simulink library "AEMS_Standard_Library"  (R2016b)
settings: Solver=ode45  StartTime=0.0  StopTime=10.0  RelTol=1e-3
undefined symbols (not defined in the file or in its folder): BkPY, carto, Cbx_extegr, Cbx_lpegrsys, Cbx_portegr, Cnx_bnk_nr_conf, Cnx_cyl_nr_conf, ConfigManagement, configuration_management, Cxx_dcm_io_tmr_end_xxxx, Cxx_dcm_rt_tmr_end, Cxx_DID_xxxx_IO_max, Cxx_DID_xxxx_IO_min, Cxx_egrhsofs, Cxx_vmaniegi, DEM_DEBOUNCE_FREEZE, DEM_DTR_CTL_INVISIBLE, DEM_DTR_CTL_NORMAL, Dem_DtrId2_XXX, Dem_DtrId3_XXX, Dem_DtrId4_XXX, Dem_DtrId5_XXX, Dem_DtrId6_XXX, Dem_DtrId7_XXX, Dem_DtrId8_XXX, Dem_DtrId9_XXX, Dem_DtrId_XXX, Dem_EnableConditionId2_XXX, Dem_EnableConditionId3_XXX, Dem_EnableConditionId4_XXX, Dem_EnableConditionId5_XXX, Dem_EnableConditionId6_XXX, Dem_EnableConditionId7_XXX, Dem_EnableConditionId8_XXX, Dem_EnableConditionId_XXX, Dem_EventId, Dem_EventId2_XXX, Dem_EventId3_XXX, Dem_EventId4_XXX, Dem_EventId5_XXX, Dem_EventId6_XXX, Dem_EventId7_XXX, Dem_EventId8_XXX, Dem_EventId9_XXX, Dem_EventId_Device_Faulttype, Dem_EventId_XXX, DEM_IUMPR_GENERAL_DENOMINATOR, DEM_OPCYC_IGNITION, Dem_RatioId2_XXX, Dem_RatioId3_XXX, Dem_RatioId4_XXX, Dem_RatioId5_XXX, Dem_RatioId6_XXX, Dem_RatioId7_XXX, Dem_RatioId8_XXX, Dem_RatioId_XXX, Dem_StorageConditionId2_XXX, Dem_StorageConditionId3_XXX, Dem_StorageConditionId4_XXX, Dem_StorageConditionId5_XXX ... (+65)
libraries: AEMS_Standard_Library x477, simulink x2
(part 35 of 39)

== system AEMS_Standard_Library/SUB/AEMS_DEM_TIME_BASED_DEBOUNCE_8D/AEMS_DEM_TIME_BASED_DEBOUNCE_CALL8 ==
  conditionfulfilled : Inport
  prefailed : Inport  Port=2
  prepassed : Inport  Port=3
  reseteventdebounce : Inport  Port=4
  DemDebounceBehavior : Inport  Port=5
  DemCounterFailedThreshold : Inport  Port=6
  DemCounterPassedThreshold : Inport  Port=7
  Enable : EnablePort
  AEMS_DEM_TIMEBASEDDEBOUNCE : AEMS_Standard_Library/SUB/AEMS_DEM_TIMEBASEDDEBOUNCE  Tag=[LIB]  eventid=Dem_EventId_Device8_Faulttype  sampletime=0.01
      settings: AttributesFormatString=|
      | %<MaskType>
      | EventId: %<eventid>
      | Sample time: %<sampletime>
  debouncevalue_for_failed : Outport
  debouncevalue_for_passed : Outport  Port=2
  failed : Outport  Port=3
  passed : Outport  Port=4
  wires:
  DemCounterPassedThreshold/1 -> AEMS_DEM_TIMEBASEDDEBOUNCE/6
  DemDebounceBehavior/1 -> AEMS_DEM_TIMEBASEDDEBOUNCE/4
  conditionfulfilled/1 -> AEMS_DEM_TIMEBASEDDEBOUNCE/1
  prepassed/1 -> AEMS_DEM_TIMEBASEDDEBOUNCE/3
  reseteventdebounce/1 -> AEMS_DEM_TIMEBASEDDEBOUNCE/7
  prefailed/1 -> AEMS_DEM_TIMEBASEDDEBOUNCE/2
  DemCounterFailedThreshold/1 -> AEMS_DEM_TIMEBASEDDEBOUNCE/5
  AEMS_DEM_TIMEBASEDDEBOUNCE/1 -> debouncevalue_for_failed/1
  AEMS_DEM_TIMEBASEDDEBOUNCE/2 -> debouncevalue_for_passed/1
  AEMS_DEM_TIMEBASEDDEBOUNCE/3 -> failed/1
  AEMS_DEM_TIMEBASEDDEBOUNCE/4 -> passed/1

== system AEMS_Standard_Library/SUB/AEMS_DEM_TIME_BASED_DEBOUNCE_THRSHOLD_DYN_1D/AEMS_DEM_TIME_BASED_DEBOUNCE_THRSHOLD_DYN_CALL ==
  conditionfulfilled : Inport
  prefailed : Inport  Port=2
  prepassed : Inport  Port=3
  reseteventdebounce : Inport  Port=4
  DemDebounceBehavior : Inport  Port=5
  DemCounterFailedThreshold : Inport  Port=6
  DemCounterPassedThreshold : Inport  Port=7
  Enable : EnablePort
      settings: AttributesFormatString=StatesWhenEnabling = %<StatesWhenEnabling>
  AEMS_DEM_TIMEBASEDDEBOUNCE : AEMS_Standard_Library/SUB/AEMS_DEM_TIMEBASEDDEBOUNCE  Tag=[LIB]  eventid=Dem_EventId_Device_Faulttype  sampletime=0.01
      settings: AttributesFormatString=|
      | %<MaskType>
      | EventId: %<eventid>
      | Sample time: %<sampletime>
  debouncevalue_for_failed : Outport
      settings: AttributesFormatString=<initial=%<InitialOutput>>\n<whendisabled=%<OutputWhenDisabled>>
  debouncevalue_for_passed : Outport  Port=2
      settings: AttributesFormatString=<initial=%<InitialOutput>>\n<whendisabled=%<OutputWhenDisabled>>
  failed : Outport  Port=3
      settings: AttributesFormatString=<initial=%<InitialOutput>>\n<whendisabled=%<OutputWhenDisabled>>
  passed : Outport  Port=4
      settings: AttributesFormatString=<initial=%<InitialOutput>>\n<whendisabled=%<OutputWhenDisabled>>
  wires:
  AEMS_DEM_TIMEBASEDDEBOUNCE/4 -> passed/1
  AEMS_DEM_TIMEBASEDDEBOUNCE/3 -> failed/1
  AEMS_DEM_TIMEBASEDDEBOUNCE/2 -> debouncevalue_for_passed/1
  AEMS_DEM_TIMEBASEDDEBOUNCE/1 -> debouncevalue_for_failed/1
  DemCounterFailedThreshold/1 -> AEMS_DEM_TIMEBASEDDEBOUNCE/5
  prefailed/1 -> AEMS_DEM_TIMEBASEDDEBOUNCE/2
  reseteventdebounce/1 -> AEMS_DEM_TIMEBASEDDEBOUNCE/7
  prepassed/1 -> AEMS_DEM_TIMEBASEDDEBOUNCE/3
  conditionfulfilled/1 -> AEMS_DEM_TIMEBASEDDEBOUNCE/1
  DemDebounceBehavior/1 -> AEMS_DEM_TIMEBASEDDEBOUNCE/4
  DemCounterPassedThreshold/1 -> AEMS_DEM_TIMEBASEDDEBOUNCE/6

== system AEMS_Standard_Library/SUB/AEMS_DEM_TIME_BASED_DEBOUNCE_THRSHOLD_DYN_2D/AEMS_DEM_TIME_BASED_DEBOUNCE_THRSHOLD_DYN_CALL1 ==
  conditionfulfilled : Inport
  prefailed : Inport  Port=2
  prepassed : Inport  Port=3
  reseteventdebounce : Inport  Port=4
  DemDebounceBehavior : Inport  Port=5
  DemCounterFailedThreshold : Inport  Port=6
  DemCounterPassedThreshold : Inport  Port=7
  Enable : EnablePort
      settings: AttributesFormatString=StatesWhenEnabling = %<StatesWhenEnabling>
  AEMS_DEM_TIMEBASEDDEBOUNCE : AEMS_Standard_Library/SUB/AEMS_DEM_TIMEBASEDDEBOUNCE  Tag=[LIB]  eventid=Dem_EventId_Device_Faulttype  sampletime=0.01
      settings: AttributesFormatString=|
      | %<MaskType>
      | EventId: %<eventid>
      | Sample time: %<sampletime>
  debouncevalue_for_failed : Outport
      settings: AttributesFormatString=<initial=%<InitialOutput>>\n<whendisabled=%<OutputWhenDisabled>>
  debouncevalue_for_passed : Outport  Port=2
      settings: AttributesFormatString=<initial=%<InitialOutput>>\n<whendisabled=%<OutputWhenDisabled>>
  failed : Outport  Port=3
      settings: AttributesFormatString=<initial=%<InitialOutput>>\n<whendisabled=%<OutputWhenDisabled>>
  passed : Outport  Port=4
      settings: AttributesFormatString=<initial=%<InitialOutput>>\n<whendisabled=%<OutputWhenDisabled>>
  wires:
  AEMS_DEM_TIMEBASEDDEBOUNCE/4 -> passed/1
  AEMS_DEM_TIMEBASEDDEBOUNCE/3 -> failed/1
  AEMS_DEM_TIMEBASEDDEBOUNCE/2 -> debouncevalue_for_passed/1
  AEMS_DEM_TIMEBASEDDEBOUNCE/1 -> debouncevalue_for_failed/1
  DemCounterFailedThreshold/1 -> AEMS_DEM_TIMEBASEDDEBOUNCE/5
  prefailed/1 -> AEMS_DEM_TIMEBASEDDEBOUNCE/2
  reseteventdebounce/1 -> AEMS_DEM_TIMEBASEDDEBOUNCE/7
  prepassed/1 -> AEMS_DEM_TIMEBASEDDEBOUNCE/3
  conditionfulfilled/1 -> AEMS_DEM_TIMEBASEDDEBOUNCE/1
  DemDebounceBehavior/1 -> AEMS_DEM_TIMEBASEDDEBOUNCE/4
  DemCounterPassedThreshold/1 -> AEMS_DEM_TIMEBASEDDEBOUNCE/6

== system AEMS_Standard_Library/SUB/AEMS_DEM_TIME_BASED_DEBOUNCE_THRSHOLD_DYN_2D/AEMS_DEM_TIME_BASED_DEBOUNCE_THRSHOLD_DYN_CALL2 ==
  conditionfulfilled : Inport
  prefailed : Inport  Port=2
  prepassed : Inport  Port=3
  reseteventdebounce : Inport  Port=4
  DemDebounceBehavior : Inport  Port=5
  DemCounterFailedThreshold : Inport  Port=6
  DemCounterPassedThreshold : Inport  Port=7
  Enable : EnablePort
      settings: AttributesFormatString=StatesWhenEnabling = %<StatesWhenEnabling>
  AEMS_DEM_TIMEBASEDDEBOUNCE : AEMS_Standard_Library/SUB/AEMS_DEM_TIMEBASEDDEBOUNCE  Tag=[LIB]  eventid=Dem_EventId_Device2_Faulttype  sampletime=0.01
      settings: AttributesFormatString=|
      | %<MaskType>
      | EventId: %<eventid>
      | Sample time: %<sampletime>
  debouncevalue_for_failed : Outport
      settings: AttributesFormatString=<initial=%<InitialOutput>>\n<whendisabled=%<OutputWhenDisabled>>
  debouncevalue_for_passed : Outport  Port=2
      settings: AttributesFormatString=<initial=%<InitialOutput>>\n<whendisabled=%<OutputWhenDisabled>>
  failed : Outport  Port=3
      settings: AttributesFormatString=<initial=%<InitialOutput>>\n<whendisabled=%<OutputWhenDisabled>>
  passed : Outport  Port=4
      settings: AttributesFormatString=<initial=%<InitialOutput>>\n<whendisabled=%<OutputWhenDisabled>>
  wires:
  DemCounterPassedThreshold/1 -> AEMS_DEM_TIMEBASEDDEBOUNCE/6
  DemDebounceBehavior/1 -> AEMS_DEM_TIMEBASEDDEBOUNCE/4
  conditionfulfilled/1 -> AEMS_DEM_TIMEBASEDDEBOUNCE/1
  prepassed/1 -> AEMS_DEM_TIMEBASEDDEBOUNCE/3
  reseteventdebounce/1 -> AEMS_DEM_TIMEBASEDDEBOUNCE/7
  prefailed/1 -> AEMS_DEM_TIMEBASEDDEBOUNCE/2
  DemCounterFailedThreshold/1 -> AEMS_DEM_TIMEBASEDDEBOUNCE/5
  AEMS_DEM_TIMEBASEDDEBOUNCE/1 -> debouncevalue_for_failed/1
  AEMS_DEM_TIMEBASEDDEBOUNCE/2 -> debouncevalue_for_passed/1
  AEMS_DEM_TIMEBASEDDEBOUNCE/3 -> failed/1
  AEMS_DEM_TIMEBASEDDEBOUNCE/4 -> passed/1

== system AEMS_Standard_Library/SUB/AEMS_DEM_TIME_BASED_DEBOUNCE_THRSHOLD_DYN_3D/AEMS_DEM_TIME_BASED_DEBOUNCE_THRSHOLD_DYN_CALL1 ==
  conditionfulfilled : Inport
  prefailed : Inport  Port=2
  prepassed : Inport  Port=3
  reseteventdebounce : Inport  Port=4
  DemDebounceBehavior : Inport  Port=5
  DemCounterFailedThreshold : Inport  Port=6
  DemCounterPassedThreshold : Inport  Port=7
  Enable : EnablePort
      settings: AttributesFormatString=StatesWhenEnabling = %<StatesWhenEnabling>
  AEMS_DEM_TIMEBASEDDEBOUNCE : AEMS_Standard_Library/SUB/AEMS_DEM_TIMEBASEDDEBOUNCE  Tag=[LIB]  eventid=Dem_EventId_Device_Faulttype  sampletime=0.01
      settings: AttributesFormatString=|
      | %<MaskType>
      | EventId: %<eventid>
      | Sample time: %<sampletime>
  debouncevalue_for_failed : Outport
      settings: AttributesFormatString=<initial=%<InitialOutput>>\n<whendisabled=%<OutputWhenDisabled>>
  debouncevalue_for_passed : Outport  Port=2
      settings: AttributesFormatString=<initial=%<InitialOutput>>\n<whendisabled=%<OutputWhenDisabled>>
  failed : Outport  Port=3
      settings: AttributesFormatString=<initial=%<InitialOutput>>\n<whendisabled=%<OutputWhenDisabled>>
  passed : Outport  Port=4
      settings: AttributesFormatString=<initial=%<InitialOutput>>\n<whendisabled=%<OutputWhenDisabled>>
  wires:
  AEMS_DEM_TIMEBASEDDEBOUNCE/4 -> passed/1
  AEMS_DEM_TIMEBASEDDEBOUNCE/3 -> failed/1
  AEMS_DEM_TIMEBASEDDEBOUNCE/2 -> debouncevalue_for_passed/1
  AEMS_DEM_TIMEBASEDDEBOUNCE/1 -> debouncevalue_for_failed/1
  DemCounterFailedThreshold/1 -> AEMS_DEM_TIMEBASEDDEBOUNCE/5
  prefailed/1 -> AEMS_DEM_TIMEBASEDDEBOUNCE/2
  reseteventdebounce/1 -> AEMS_DEM_TIMEBASEDDEBOUNCE/7
  prepassed/1 -> AEMS_DEM_TIMEBASEDDEBOUNCE/3
  conditionfulfilled/1 -> AEMS_DEM_TIMEBASEDDEBOUNCE/1
  DemDebounceBehavior/1 -> AEMS_DEM_TIMEBASEDDEBOUNCE/4
  DemCounterPassedThreshold/1 -> AEMS_DEM_TIMEBASEDDEBOUNCE/6

== system AEMS_Standard_Library/SUB/AEMS_DEM_TIME_BASED_DEBOUNCE_THRSHOLD_DYN_3D/AEMS_DEM_TIME_BASED_DEBOUNCE_THRSHOLD_DYN_CALL2 ==
  conditionfulfilled : Inport
  prefailed : Inport  Port=2
  prepassed : Inport  Port=3
  reseteventdebounce : Inport  Port=4
  DemDebounceBehavior : Inport  Port=5
  DemCounterFailedThreshold : Inport  Port=6
  DemCounterPassedThreshold : Inport  Port=7
  Enable : EnablePort
      settings: AttributesFormatString=StatesWhenEnabling = %<StatesWhenEnabling>
  AEMS_DEM_TIMEBASEDDEBOUNCE : AEMS_Standard_Library/SUB/AEMS_DEM_TIMEBASEDDEBOUNCE  Tag=[LIB]  eventid=Dem_EventId_Device2_Faulttype  sampletime=0.01
      settings: AttributesFormatString=|
      | %<MaskType>
      | EventId: %<eventid>
      | Sample time: %<sampletime>
  debouncevalue_for_failed : Outport
      settings: AttributesFormatString=<initial=%<InitialOutput>>\n<whendisabled=%<OutputWhenDisabled>>
  debouncevalue_for_passed : Outport  Port=2
      settings: AttributesFormatString=<initial=%<InitialOutput>>\n<whendisabled=%<OutputWhenDisabled>>
  failed : Outport  Port=3
      settings: AttributesFormatString=<initial=%<InitialOutput>>\n<whendisabled=%<OutputWhenDisabled>>
  passed : Outport  Port=4
      settings: AttributesFormatString=<initial=%<InitialOutput>>\n<whendisabled=%<OutputWhenDisabled>>
  wires:
  DemCounterPassedThreshold/1 -> AEMS_DEM_TIMEBASEDDEBOUNCE/6
  DemDebounceBehavior/1 -> AEMS_DEM_TIMEBASEDDEBOUNCE/4
  conditionfulfilled/1 -> AEMS_DEM_TIMEBASEDDEBOUNCE/1
  prepassed/1 -> AEMS_DEM_TIMEBASEDDEBOUNCE/3
  reseteventdebounce/1 -> AEMS_DEM_TIMEBASEDDEBOUNCE/7
  prefailed/1 -> AEMS_DEM_TIMEBASEDDEBOUNCE/2
  DemCounterFailedThreshold/1 -> AEMS_DEM_TIMEBASEDDEBOUNCE/5
  AEMS_DEM_TIMEBASEDDEBOUNCE/1 -> debouncevalue_for_failed/1
  AEMS_DEM_TIMEBASEDDEBOUNCE/2 -> debouncevalue_for_passed/1
  AEMS_DEM_TIMEBASEDDEBOUNCE/3 -> failed/1
  AEMS_DEM_TIMEBASEDDEBOUNCE/4 -> passed/1

== system AEMS_Standard_Library/SUB/AEMS_DEM_TIME_BASED_DEBOUNCE_THRSHOLD_DYN_3D/AEMS_DEM_TIME_BASED_DEBOUNCE_THRSHOLD_DYN_CALL3 ==
  conditionfulfilled : Inport
  prefailed : Inport  Port=2
  prepassed : Inport  Port=3
  reseteventdebounce : Inport  Port=4
  DemDebounceBehavior : Inport  Port=5
  DemCounterFailedThreshold : Inport  Port=6
  DemCounterPassedThreshold : Inport  Port=7
  Enable : EnablePort
      settings: AttributesFormatString=StatesWhenEnabling = %<StatesWhenEnabling>
  AEMS_DEM_TIMEBASEDDEBOUNCE : AEMS_Standard_Library/SUB/AEMS_DEM_TIMEBASEDDEBOUNCE  Tag=[LIB]  eventid=Dem_EventId_Device3_Faulttype  sampletime=0.01
      settings: AttributesFormatString=|
      | %<MaskType>
      | EventId: %<eventid>
      | Sample time: %<sampletime>
  debouncevalue_for_failed : Outport
      settings: AttributesFormatString=<initial=%<InitialOutput>>\n<whendisabled=%<OutputWhenDisabled>>
  debouncevalue_for_passed : Outport  Port=2
      settings: AttributesFormatString=<initial=%<InitialOutput>>\n<whendisabled=%<OutputWhenDisabled>>
  failed : Outport  Port=3
      settings: AttributesFormatString=<initial=%<InitialOutput>>\n<whendisabled=%<OutputWhenDisabled>>
  passed : Outport  Port=4
      settings: AttributesFormatString=<initial=%<InitialOutput>>\n<whendisabled=%<OutputWhenDisabled>>
  wires:
  DemCounterPassedThreshold/1 -> AEMS_DEM_TIMEBASEDDEBOUNCE/6
  DemDebounceBehavior/1 -> AEMS_DEM_TIMEBASEDDEBOUNCE/4
  conditionfulfilled/1 -> AEMS_DEM_TIMEBASEDDEBOUNCE/1
  prepassed/1 -> AEMS_DEM_TIMEBASEDDEBOUNCE/3
  reseteventdebounce/1 -> AEMS_DEM_TIMEBASEDDEBOUNCE/7
  prefailed/1 -> AEMS_DEM_TIMEBASEDDEBOUNCE/2
  DemCounterFailedThreshold/1 -> AEMS_DEM_TIMEBASEDDEBOUNCE/5
  AEMS_DEM_TIMEBASEDDEBOUNCE/1 -> debouncevalue_for_failed/1
  AEMS_DEM_TIMEBASEDDEBOUNCE/2 -> debouncevalue_for_passed/1
  AEMS_DEM_TIMEBASEDDEBOUNCE/3 -> failed/1
  AEMS_DEM_TIMEBASEDDEBOUNCE/4 -> passed/1

== system AEMS_Standard_Library/SUB/AEMS_DEM_TIME_BASED_DEBOUNCE_THRSHOLD_DYN_4D/AEMS_DEM_TIME_BASED_DEBOUNCE_THRSHOLD_DYN_CALL1 ==
  conditionfulfilled : Inport
  prefailed : Inport  Port=2
  prepassed : Inport  Port=3
  reseteventdebounce : Inport  Port=4
  DemDebounceBehavior : Inport  Port=5
  DemCounterFailedThreshold : Inport  Port=6
  DemCounterPassedThreshold : Inport  Port=7
  Enable : EnablePort
      settings: AttributesFormatString=StatesWhenEnabling = %<StatesWhenEnabling>
  AEMS_DEM_TIMEBASEDDEBOUNCE : AEMS_Standard_Library/SUB/AEMS_DEM_TIMEBASEDDEBOUNCE  Tag=[LIB]  eventid=Dem_EventId_Device_Faulttype  sampletime=0.01
      settings: AttributesFormatString=|
      | %<MaskType>
      | EventId: %<eventid>
      | Sample time: %<sampletime>
  debouncevalue_for_failed : Outport
      settings: AttributesFormatString=<initial=%<InitialOutput>>\n<whendisabled=%<OutputWhenDisabled>>
  debouncevalue_for_passed : Outport  Port=2
      settings: AttributesFormatString=<initial=%<InitialOutput>>\n<whendisabled=%<OutputWhenDisabled>>
  failed : Outport  Port=3
      settings: AttributesFormatString=<initial=%<InitialOutput>>\n<whendisabled=%<OutputWhenDisabled>>
  passed : Outport  Port=4
      settings: AttributesFormatString=<initial=%<InitialOutput>>\n<whendisabled=%<OutputWhenDisabled>>
  wires:
  AEMS_DEM_TIMEBASEDDEBOUNCE/4 -> passed/1
  AEMS_DEM_TIMEBASEDDEBOUNCE/3 -> failed/1
  AEMS_DEM_TIMEBASEDDEBOUNCE/2 -> debouncevalue_for_passed/1
  AEMS_DEM_TIMEBASEDDEBOUNCE/1 -> debouncevalue_for_failed/1
  DemCounterFailedThreshold/1 -> AEMS_DEM_TIMEBASEDDEBOUNCE/5
  prefailed/1 -> AEMS_DEM_TIMEBASEDDEBOUNCE/2
  reseteventdebounce/1 -> AEMS_DEM_TIMEBASEDDEBOUNCE/7
  prepassed/1 -> AEMS_DEM_TIMEBASEDDEBOUNCE/3
  conditionfulfilled/1 -> AEMS_DEM_TIMEBASEDDEBOUNCE/1
  DemDebounceBehavior/1 -> AEMS_DEM_TIMEBASEDDEBOUNCE/4
  DemCounterPassedThreshold/1 -> AEMS_DEM_TIMEBASEDDEBOUNCE/6

== system AEMS_Standard_Library/SUB/AEMS_DEM_TIME_BASED_DEBOUNCE_THRSHOLD_DYN_4D/AEMS_DEM_TIME_BASED_DEBOUNCE_THRSHOLD_DYN_CALL2 ==
  conditionfulfilled : Inport
  prefailed : Inport  Port=2
  prepassed : Inport  Port=3
  reseteventdebounce : Inport  Port=4
  DemDebounceBehavior : Inport  Port=5
  DemCounterFailedThreshold : Inport  Port=6
  DemCounterPassedThreshold : Inport  Port=7
  Enable : EnablePort
      settings: AttributesFormatString=StatesWhenEnabling = %<StatesWhenEnabling>
  AEMS_DEM_TIMEBASEDDEBOUNCE : AEMS_Standard_Library/SUB/AEMS_DEM_TIMEBASEDDEBOUNCE  Tag=[LIB]  eventid=Dem_EventId_Device2_Faulttype  sampletime=0.01
      settings: AttributesFormatString=|
      | %<MaskType>
      | EventId: %<eventid>
      | Sample time: %<sampletime>
  debouncevalue_for_failed : Outport
      settings: AttributesFormatString=<initial=%<InitialOutput>>\n<whendisabled=%<OutputWhenDisabled>>
  debouncevalue_for_passed : Outport  Port=2
      settings: AttributesFormatString=<initial=%<InitialOutput>>\n<whendisabled=%<OutputWhenDisabled>>
  failed : Outport  Port=3
      settings: AttributesFormatString=<initial=%<InitialOutput>>\n<whendisabled=%<OutputWhenDisabled>>
  passed : Outport  Port=4
      settings: AttributesFormatString=<initial=%<InitialOutput>>\n<whendisabled=%<OutputWhenDisabled>>
  wires:
  DemCounterPassedThreshold/1 -> AEMS_DEM_TIMEBASEDDEBOUNCE/6
  DemDebounceBehavior/1 -> AEMS_DEM_TIMEBASEDDEBOUNCE/4
  conditionfulfilled/1 -> AEMS_DEM_TIMEBASEDDEBOUNCE/1
  prepassed/1 -> AEMS_DEM_TIMEBASEDDEBOUNCE/3
  reseteventdebounce/1 -> AEMS_DEM_TIMEBASEDDEBOUNCE/7
  prefailed/1 -> AEMS_DEM_TIMEBASEDDEBOUNCE/2
  DemCounterFailedThreshold/1 -> AEMS_DEM_TIMEBASEDDEBOUNCE/5
  AEMS_DEM_TIMEBASEDDEBOUNCE/1 -> debouncevalue_for_failed/1
  AEMS_DEM_TIMEBASEDDEBOUNCE/2 -> debouncevalue_for_passed/1
  AEMS_DEM_TIMEBASEDDEBOUNCE/3 -> failed/1
  AEMS_DEM_TIMEBASEDDEBOUNCE/4 -> passed/1

== system AEMS_Standard_Library/SUB/AEMS_DEM_TIME_BASED_DEBOUNCE_THRSHOLD_DYN_4D/AEMS_DEM_TIME_BASED_DEBOUNCE_THRSHOLD_DYN_CALL3 ==
  conditionfulfilled : Inport
  prefailed : Inport  Port=2
  prepassed : Inport  Port=3
  reseteventdebounce : Inport  Port=4
  DemDebounceBehavior : Inport  Port=5
  DemCounterFailedThreshold : Inport  Port=6
  DemCounterPassedThreshold : Inport  Port=7
  Enable : EnablePort
      settings: AttributesFormatString=StatesWhenEnabling = %<StatesWhenEnabling>
  AEMS_DEM_TIMEBASEDDEBOUNCE : AEMS_Standard_Library/SUB/AEMS_DEM_TIMEBASEDDEBOUNCE  Tag=[LIB]  eventid=Dem_EventId_Device3_Faulttype  sampletime=0.01
      settings: AttributesFormatString=|
      | %<MaskType>
      | EventId: %<eventid>
      | Sample time: %<sampletime>
  debouncevalue_for_failed : Outport
      settings: AttributesFormatString=<initial=%<InitialOutput>>\n<whendisabled=%<OutputWhenDisabled>>
  debouncevalue_for_passed : Outport  Port=2
      settings: AttributesFormatString=<initial=%<InitialOutput>>\n<whendisabled=%<OutputWhenDisabled>>
  failed : Outport  Port=3
      settings: AttributesFormatString=<initial=%<InitialOutput>>\n<whendisabled=%<OutputWhenDisabled>>
  passed : Outport  Port=4
      settings: AttributesFormatString=<initial=%<InitialOutput>>\n<whendisabled=%<OutputWhenDisabled>>
  wires:
  DemCounterPassedThreshold/1 -> AEMS_DEM_TIMEBASEDDEBOUNCE/6
  DemDebounceBehavior/1 -> AEMS_DEM_TIMEBASEDDEBOUNCE/4
  conditionfulfilled/1 -> AEMS_DEM_TIMEBASEDDEBOUNCE/1
  prepassed/1 -> AEMS_DEM_TIMEBASEDDEBOUNCE/3
  reseteventdebounce/1 -> AEMS_DEM_TIMEBASEDDEBOUNCE/7
  prefailed/1 -> AEMS_DEM_TIMEBASEDDEBOUNCE/2
  DemCounterFailedThreshold/1 -> AEMS_DEM_TIMEBASEDDEBOUNCE/5
  AEMS_DEM_TIMEBASEDDEBOUNCE/1 -> debouncevalue_for_failed/1
  AEMS_DEM_TIMEBASEDDEBOUNCE/2 -> debouncevalue_for_passed/1
  AEMS_DEM_TIMEBASEDDEBOUNCE/3 -> failed/1
  AEMS_DEM_TIMEBASEDDEBOUNCE/4 -> passed/1

== system AEMS_Standard_Library/SUB/AEMS_DEM_TIME_BASED_DEBOUNCE_THRSHOLD_DYN_4D/AEMS_DEM_TIME_BASED_DEBOUNCE_THRSHOLD_DYN_CALL4 ==
  conditionfulfilled : Inport
  prefailed : Inport  Port=2
  prepassed : Inport  Port=3
  reseteventdebounce : Inport  Port=4
  DemDebounceBehavior : Inport  Port=5
  DemCounterFailedThreshold : Inport  Port=6
  DemCounterPassedThreshold : Inport  Port=7
  Enable : EnablePort
      settings: AttributesFormatString=StatesWhenEnabling = %<StatesWhenEnabling>
  AEMS_DEM_TIMEBASEDDEBOUNCE : AEMS_Standard_Library/SUB/AEMS_DEM_TIMEBASEDDEBOUNCE  Tag=[LIB]  eventid=Dem_EventId_Device4_Faulttype  sampletime=0.01
      settings: AttributesFormatString=|
      | %<MaskType>
      | EventId: %<eventid>
      | Sample time: %<sampletime>
  debouncevalue_for_failed : Outport
      settings: AttributesFormatString=<initial=%<InitialOutput>>\n<whendisabled=%<OutputWhenDisabled>>
  debouncevalue_for_passed : Outport  Port=2
      settings: AttributesFormatString=<initial=%<InitialOutput>>\n<whendisabled=%<OutputWhenDisabled>>
  failed : Outport  Port=3
      settings: AttributesFormatString=<initial=%<InitialOutput>>\n<whendisabled=%<OutputWhenDisabled>>
  passed : Outport  Port=4
      settings: AttributesFormatString=<initial=%<InitialOutput>>\n<whendisabled=%<OutputWhenDisabled>>
  wires:
  DemCounterPassedThreshold/1 -> AEMS_DEM_TIMEBASEDDEBOUNCE/6
  DemDebounceBehavior/1 -> AEMS_DEM_TIMEBASEDDEBOUNCE/4
  conditionfulfilled/1 -> AEMS_DEM_TIMEBASEDDEBOUNCE/1
  prepassed/1 -> AEMS_DEM_TIMEBASEDDEBOUNCE/3
  reseteventdebounce/1 -> AEMS_DEM_TIMEBASEDDEBOUNCE/7
  prefailed/1 -> AEMS_DEM_TIMEBASEDDEBOUNCE/2
  DemCounterFailedThreshold/1 -> AEMS_DEM_TIMEBASEDDEBOUNCE/5
  AEMS_DEM_TIMEBASEDDEBOUNCE/1 -> debouncevalue_for_failed/1
  AEMS_DEM_TIMEBASEDDEBOUNCE/2 -> debouncevalue_for_passed/1
  AEMS_DEM_TIMEBASEDDEBOUNCE/3 -> failed/1
  AEMS_DEM_TIMEBASEDDEBOUNCE/4 -> passed/1

== system AEMS_Standard_Library/SUB/AEMS_DEM_TIME_BASED_DEBOUNCE_THRSHOLD_DYN_6D/AEMS_DEM_TIME_BASED_DEBOUNCE_THRSHOLD_DYN_CALL1 ==
  conditionfulfilled : Inport
  prefailed : Inport  Port=2
  prepassed : Inport  Port=3
  reseteventdebounce : Inport  Port=4
  DemDebounceBehavior : Inport  Port=5
  DemCounterFailedThreshold : Inport  Port=6
  DemCounterPassedThreshold : Inport  Port=7
  Enable : EnablePort
      settings: AttributesFormatString=StatesWhenEnabling = %<StatesWhenEnabling>
  AEMS_DEM_TIMEBASEDDEBOUNCE : AEMS_Standard_Library/SUB/AEMS_DEM_TIMEBASEDDEBOUNCE  Tag=[LIB]  eventid=Dem_EventId_Device_Faulttype  sampletime=0.01
      settings: AttributesFormatString=|
      | %<MaskType>
      | EventId: %<eventid>
      | Sample time: %<sampletime>
  debouncevalue_for_failed : Outport
      settings: AttributesFormatString=<initial=%<InitialOutput>>\n<whendisabled=%<OutputWhenDisabled>>
  debouncevalue_for_passed : Outport  Port=2
      settings: AttributesFormatString=<initial=%<InitialOutput>>\n<whendisabled=%<OutputWhenDisabled>>
  failed : Outport  Port=3
      settings: AttributesFormatString=<initial=%<InitialOutput>>\n<whendisabled=%<OutputWhenDisabled>>
  passed : Outport  Port=4
      settings: AttributesFormatString=<initial=%<InitialOutput>>\n<whendisabled=%<OutputWhenDisabled>>
  wires:
  DemCounterPassedThreshold/1 -> AEMS_DEM_TIMEBASEDDEBOUNCE/6
  DemDebounceBehavior/1 -> AEMS_DEM_TIMEBASEDDEBOUNCE/4
  conditionfulfilled/1 -> AEMS_DEM_TIMEBASEDDEBOUNCE/1
  prepassed/1 -> AEMS_DEM_TIMEBASEDDEBOUNCE/3
  reseteventdebounce/1 -> AEMS_DEM_TIMEBASEDDEBOUNCE/7
  prefailed/1 -> AEMS_DEM_TIMEBASEDDEBOUNCE/2
  DemCounterFailedThreshold/1 -> AEMS_DEM_TIMEBASEDDEBOUNCE/5
  AEMS_DEM_TIMEBASEDDEBOUNCE/1 -> debouncevalue_for_failed/1
  AEMS_DEM_TIMEBASEDDEBOUNCE/2 -> debouncevalue_for_passed/1
  AEMS_DEM_TIMEBASEDDEBOUNCE/3 -> failed/1
  AEMS_DEM_TIMEBASEDDEBOUNCE/4 -> passed/1

== system AEMS_Standard_Library/SUB/AEMS_DEM_TIME_BASED_DEBOUNCE_THRSHOLD_DYN_6D/AEMS_DEM_TIME_BASED_DEBOUNCE_THRSHOLD_DYN_CALL2 ==
  conditionfulfilled : Inport
  prefailed : Inport  Port=2
  prepassed : Inport  Port=3
  reseteventdebounce : Inport  Port=4
  DemDebounceBehavior : Inport  Port=5
  DemCounterFailedThreshold : Inport  Port=6
  DemCounterPassedThreshold : Inport  Port=7
  Enable : EnablePort
      settings: AttributesFormatString=StatesWhenEnabling = %<StatesWhenEnabling>
  AEMS_DEM_TIMEBASEDDEBOUNCE : AEMS_Standard_Library/SUB/AEMS_DEM_TIMEBASEDDEBOUNCE  Tag=[LIB]  eventid=Dem_EventId_Device2_Faulttype  sampletime=0.01
      settings: AttributesFormatString=|
      | %<MaskType>
      | EventId: %<eventid>
      | Sample time: %<sampletime>
  debouncevalue_for_failed : Outport
      settings: AttributesFormatString=<initial=%<InitialOutput>>\n<whendisabled=%<OutputWhenDisabled>>
  debouncevalue_for_passed : Outport  Port=2
      settings: AttributesFormatString=<initial=%<InitialOutput>>\n<whendisabled=%<OutputWhenDisabled>>
  failed : Outport  Port=3
      settings: AttributesFormatString=<initial=%<InitialOutput>>\n<whendisabled=%<OutputWhenDisabled>>
  passed : Outport  Port=4
      settings: AttributesFormatString=<initial=%<InitialOutput>>\n<whendisabled=%<OutputWhenDisabled>>
  wires:
  AEMS_DEM_TIMEBASEDDEBOUNCE/4 -> passed/1
  AEMS_DEM_TIMEBASEDDEBOUNCE/3 -> failed/1
  AEMS_DEM_TIMEBASEDDEBOUNCE/2 -> debouncevalue_for_passed/1
  AEMS_DEM_TIMEBASEDDEBOUNCE/1 -> debouncevalue_for_failed/1
  DemCounterFailedThreshold/1 -> AEMS_DEM_TIMEBASEDDEBOUNCE/5
  prefailed/1 -> AEMS_DEM_TIMEBASEDDEBOUNCE/2
  reseteventdebounce/1 -> AEMS_DEM_TIMEBASEDDEBOUNCE/7
  prepassed/1 -> AEMS_DEM_TIMEBASEDDEBOUNCE/3
  conditionfulfilled/1 -> AEMS_DEM_TIMEBASEDDEBOUNCE/1
  DemDebounceBehavior/1 -> AEMS_DEM_TIMEBASEDDEBOUNCE/4
  DemCounterPassedThreshold/1 -> AEMS_DEM_TIMEBASEDDEBOUNCE/6

== system AEMS_Standard_Library/SUB/AEMS_DEM_TIME_BASED_DEBOUNCE_THRSHOLD_DYN_6D/AEMS_DEM_TIME_BASED_DEBOUNCE_THRSHOLD_DYN_CALL3 ==
  conditionfulfilled : Inport
  prefailed : Inport  Port=2
  prepassed : Inport  Port=3
  reseteventdebounce : Inport  Port=4
  DemDebounceBehavior : Inport  Port=5
  DemCounterFailedThreshold : Inport  Port=6
  DemCounterPassedThreshold : Inport  Port=7
  Enable : EnablePort
      settings: AttributesFormatString=StatesWhenEnabling = %<StatesWhenEnabling>
  AEMS_DEM_TIMEBASEDDEBOUNCE : AEMS_Standard_Library/SUB/AEMS_DEM_TIMEBASEDDEBOUNCE  Tag=[LIB]  eventid=Dem_EventId_Device3_Faulttype  sampletime=0.01
      settings: AttributesFormatString=|
      | %<MaskType>
      | EventId: %<eventid>
      | Sample time: %<sampletime>
  debouncevalue_for_failed : Outport
      settings: AttributesFormatString=<initial=%<InitialOutput>>\n<whendisabled=%<OutputWhenDisabled>>
  debouncevalue_for_passed : Outport  Port=2
      settings: AttributesFormatString=<initial=%<InitialOutput>>\n<whendisabled=%<OutputWhenDisabled>>
  failed : Outport  Port=3
      settings: AttributesFormatString=<initial=%<InitialOutput>>\n<whendisabled=%<OutputWhenDisabled>>
  passed : Outport  Port=4
      settings: AttributesFormatString=<initial=%<InitialOutput>>\n<whendisabled=%<OutputWhenDisabled>>
  wires:
  AEMS_DEM_TIMEBASEDDEBOUNCE/4 -> passed/1
  AEMS_DEM_TIMEBASEDDEBOUNCE/3 -> failed/1
  AEMS_DEM_TIMEBASEDDEBOUNCE/2 -> debouncevalue_for_passed/1
  AEMS_DEM_TIMEBASEDDEBOUNCE/1 -> debouncevalue_for_failed/1
  DemCounterFailedThreshold/1 -> AEMS_DEM_TIMEBASEDDEBOUNCE/5
  prefailed/1 -> AEMS_DEM_TIMEBASEDDEBOUNCE/2
  reseteventdebounce/1 -> AEMS_DEM_TIMEBASEDDEBOUNCE/7
  prepassed/1 -> AEMS_DEM_TIMEBASEDDEBOUNCE/3
  conditionfulfilled/1 -> AEMS_DEM_TIMEBASEDDEBOUNCE/1
  DemDebounceBehavior/1 -> AEMS_DEM_TIMEBASEDDEBOUNCE/4
  DemCounterPassedThreshold/1 -> AEMS_DEM_TIMEBASEDDEBOUNCE/6

== system AEMS_Standard_Library/SUB/AEMS_DEM_TIME_BASED_DEBOUNCE_THRSHOLD_DYN_6D/AEMS_DEM_TIME_BASED_DEBOUNCE_THRSHOLD_DYN_CALL4 ==
  conditionfulfilled : Inport
  prefailed : Inport  Port=2
  prepassed : Inport  Port=3
  reseteventdebounce : Inport  Port=4
  DemDebounceBehavior : Inport  Port=5
  DemCounterFailedThreshold : Inport  Port=6
  DemCounterPassedThreshold : Inport  Port=7
  Enable : EnablePort
      settings: AttributesFormatString=StatesWhenEnabling = %<StatesWhenEnabling>
  AEMS_DEM_TIMEBASEDDEBOUNCE : AEMS_Standard_Library/SUB/AEMS_DEM_TIMEBASEDDEBOUNCE  Tag=[LIB]  eventid=Dem_EventId_Device4_Faulttype  sampletime=0.01
      settings: AttributesFormatString=|
      | %<MaskType>
      | EventId: %<eventid>
      | Sample time: %<sampletime>
  debouncevalue_for_failed : Outport
      settings: AttributesFormatString=<initial=%<InitialOutput>>\n<whendisabled=%<OutputWhenDisabled>>
  debouncevalue_for_passed : Outport  Port=2
      settings: AttributesFormatString=<initial=%<InitialOutput>>\n<whendisabled=%<OutputWhenDisabled>>
  failed : Outport  Port=3
      settings: AttributesFormatString=<initial=%<InitialOutput>>\n<whendisabled=%<OutputWhenDisabled>>
  passed : Outport  Port=4
      settings: AttributesFormatString=<initial=%<InitialOutput>>\n<whendisabled=%<OutputWhenDisabled>>
  wires:
  AEMS_DEM_TIMEBASEDDEBOUNCE/4 -> passed/1
  AEMS_DEM_TIMEBASEDDEBOUNCE/3 -> failed/1
  AEMS_DEM_TIMEBASEDDEBOUNCE/2 -> debouncevalue_for_passed/1
  AEMS_DEM_TIMEBASEDDEBOUNCE/1 -> debouncevalue_for_failed/1
  DemCounterFailedThreshold/1 -> AEMS_DEM_TIMEBASEDDEBOUNCE/5
  prefailed/1 -> AEMS_DEM_TIMEBASEDDEBOUNCE/2
  reseteventdebounce/1 -> AEMS_DEM_TIMEBASEDDEBOUNCE/7
  prepassed/1 -> AEMS_DEM_TIMEBASEDDEBOUNCE/3
  conditionfulfilled/1 -> AEMS_DEM_TIMEBASEDDEBOUNCE/1
  DemDebounceBehavior/1 -> AEMS_DEM_TIMEBASEDDEBOUNCE/4
  DemCounterPassedThreshold/1 -> AEMS_DEM_TIMEBASEDDEBOUNCE/6

== system AEMS_Standard_Library/SUB/AEMS_DEM_TIME_BASED_DEBOUNCE_THRSHOLD_DYN_6D/AEMS_DEM_TIME_BASED_DEBOUNCE_THRSHOLD_DYN_CALL5 ==
  conditionfulfilled : Inport
  prefailed : Inport  Port=2
  prepassed : Inport  Port=3
  reseteventdebounce : Inport  Port=4
  DemDebounceBehavior : Inport  Port=5
  DemCounterFailedThreshold : Inport  Port=6
  DemCounterPassedThreshold : Inport  Port=7
  Enable : EnablePort
      settings: AttributesFormatString=StatesWhenEnabling = %<StatesWhenEnabling>
  AEMS_DEM_TIMEBASEDDEBOUNCE : AEMS_Standard_Library/SUB/AEMS_DEM_TIMEBASEDDEBOUNCE  Tag=[LIB]  eventid=Dem_EventId_Device5_Faulttype  sampletime=0.01
      settings: AttributesFormatString=|
      | %<MaskType>
      | EventId: %<eventid>
      | Sample time: %<sampletime>
  debouncevalue_for_failed : Outport
      settings: AttributesFormatString=<initial=%<InitialOutput>>\n<whendisabled=%<OutputWhenDisabled>>
  debouncevalue_for_passed : Outport  Port=2
      settings: AttributesFormatString=<initial=%<InitialOutput>>\n<whendisabled=%<OutputWhenDisabled>>
  failed : Outport  Port=3
      settings: AttributesFormatString=<initial=%<InitialOutput>>\n<whendisabled=%<OutputWhenDisabled>>
  passed : Outport  Port=4
      settings: AttributesFormatString=<initial=%<InitialOutput>>\n<whendisabled=%<OutputWhenDisabled>>
  wires:
  AEMS_DEM_TIMEBASEDDEBOUNCE/4 -> passed/1
  AEMS_DEM_TIMEBASEDDEBOUNCE/3 -> failed/1
  AEMS_DEM_TIMEBASEDDEBOUNCE/2 -> debouncevalue_for_passed/1
  AEMS_DEM_TIMEBASEDDEBOUNCE/1 -> debouncevalue_for_failed/1
  DemCounterFailedThreshold/1 -> AEMS_DEM_TIMEBASEDDEBOUNCE/5
  prefailed/1 -> AEMS_DEM_TIMEBASEDDEBOUNCE/2
  reseteventdebounce/1 -> AEMS_DEM_TIMEBASEDDEBOUNCE/7
  prepassed/1 -> AEMS_DEM_TIMEBASEDDEBOUNCE/3
  conditionfulfilled/1 -> AEMS_DEM_TIMEBASEDDEBOUNCE/1
  DemDebounceBehavior/1 -> AEMS_DEM_TIMEBASEDDEBOUNCE/4
  DemCounterPassedThreshold/1 -> AEMS_DEM_TIMEBASEDDEBOUNCE/6

== system AEMS_Standard_Library/SUB/AEMS_DEM_TIME_BASED_DEBOUNCE_THRSHOLD_DYN_6D/AEMS_DEM_TIME_BASED_DEBOUNCE_THRSHOLD_DYN_CALL6 ==
  conditionfulfilled : Inport
  prefailed : Inport  Port=2
  prepassed : Inport  Port=3
  reseteventdebounce : Inport  Port=4
  DemDebounceBehavior : Inport  Port=5
  DemCounterFailedThreshold : Inport  Port=6
  DemCounterPassedThreshold : Inport  Port=7
  Enable : EnablePort
      settings: AttributesFormatString=StatesWhenEnabling = %<StatesWhenEnabling>
  AEMS_DEM_TIMEBASEDDEBOUNCE : AEMS_Standard_Library/SUB/AEMS_DEM_TIMEBASEDDEBOUNCE  Tag=[LIB]  eventid=Dem_EventId_Device6_Faulttype  sampletime=0.01
      settings: AttributesFormatString=|
      | %<MaskType>
      | EventId: %<eventid>
      | Sample time: %<sampletime>
  debouncevalue_for_failed : Outport
      settings: AttributesFormatString=<initial=%<InitialOutput>>\n<whendisabled=%<OutputWhenDisabled>>
  debouncevalue_for_passed : Outport  Port=2
      settings: AttributesFormatString=<initial=%<InitialOutput>>\n<whendisabled=%<OutputWhenDisabled>>
  failed : Outport  Port=3
      settings: AttributesFormatString=<initial=%<InitialOutput>>\n<whendisabled=%<OutputWhenDisabled>>
  passed : Outport  Port=4
      settings: AttributesFormatString=<initial=%<InitialOutput>>\n<whendisabled=%<OutputWhenDisabled>>
  wires:
  AEMS_DEM_TIMEBASEDDEBOUNCE/4 -> passed/1
  AEMS_DEM_TIMEBASEDDEBOUNCE/3 -> failed/1
  AEMS_DEM_TIMEBASEDDEBOUNCE/2 -> debouncevalue_for_passed/1
  AEMS_DEM_TIMEBASEDDEBOUNCE/1 -> debouncevalue_for_failed/1
  DemCounterFailedThreshold/1 -> AEMS_DEM_TIMEBASEDDEBOUNCE/5
  prefailed/1 -> AEMS_DEM_TIMEBASEDDEBOUNCE/2
  reseteventdebounce/1 -> AEMS_DEM_TIMEBASEDDEBOUNCE/7
  prepassed/1 -> AEMS_DEM_TIMEBASEDDEBOUNCE/3
  conditionfulfilled/1 -> AEMS_DEM_TIMEBASEDDEBOUNCE/1
  DemDebounceBehavior/1 -> AEMS_DEM_TIMEBASEDDEBOUNCE/4
  DemCounterPassedThreshold/1 -> AEMS_DEM_TIMEBASEDDEBOUNCE/6

== system AEMS_Standard_Library/SUB/AEMS_DEM_TIME_BASED_DEBOUNCE_THRSHOLD_DYN_8D/AEMS_DEM_TIME_BASED_DEBOUNCE_THRSHOLD_DYN_CALL1 ==
  conditionfulfilled : Inport
  prefailed : Inport  Port=2
  prepassed : Inport  Port=3
  reseteventdebounce : Inport  Port=4
  DemDebounceBehavior : Inport  Port=5
  DemCounterFailedThreshold : Inport  Port=6
  DemCounterPassedThreshold : Inport  Port=7
  Enable : EnablePort
      settings: AttributesFormatString=StatesWhenEnabling = %<StatesWhenEnabling>
  AEMS_DEM_TIMEBASEDDEBOUNCE : AEMS_Standard_Library/SUB/AEMS_DEM_TIMEBASEDDEBOUNCE  Tag=[LIB]  eventid=Dem_EventId_Device_Faulttype  sampletime=0.01
      settings: AttributesFormatString=|
      | %<MaskType>
      | EventId: %<eventid>
      | Sample time: %<sampletime>
  debouncevalue_for_failed : Outport
      settings: AttributesFormatString=<initial=%<InitialOutput>>\n<whendisabled=%<OutputWhenDisabled>>
  debouncevalue_for_passed : Outport  Port=2
      settings: AttributesFormatString=<initial=%<InitialOutput>>\n<whendisabled=%<OutputWhenDisabled>>
  failed : Outport  Port=3
      settings: AttributesFormatString=<initial=%<InitialOutput>>\n<whendisabled=%<OutputWhenDisabled>>
  passed : Outport  Port=4
      settings: AttributesFormatString=<initial=%<InitialOutput>>\n<whendisabled=%<OutputWhenDisabled>>
  wires:
  DemCounterPassedThreshold/1 -> AEMS_DEM_TIMEBASEDDEBOUNCE/6
  DemDebounceBehavior/1 -> AEMS_DEM_TIMEBASEDDEBOUNCE/4
  conditionfulfilled/1 -> AEMS_DEM_TIMEBASEDDEBOUNCE/1
  prepassed/1 -> AEMS_DEM_TIMEBASEDDEBOUNCE/3
  reseteventdebounce/1 -> AEMS_DEM_TIMEBASEDDEBOUNCE/7
  prefailed/1 -> AEMS_DEM_TIMEBASEDDEBOUNCE/2
  DemCounterFailedThreshold/1 -> AEMS_DEM_TIMEBASEDDEBOUNCE/5
  AEMS_DEM_TIMEBASEDDEBOUNCE/1 -> debouncevalue_for_failed/1
  AEMS_DEM_TIMEBASEDDEBOUNCE/2 -> debouncevalue_for_passed/1
  AEMS_DEM_TIMEBASEDDEBOUNCE/3 -> failed/1
  AEMS_DEM_TIMEBASEDDEBOUNCE/4 -> passed/1

== system AEMS_Standard_Library/SUB/AEMS_DEM_TIME_BASED_DEBOUNCE_THRSHOLD_DYN_8D/AEMS_DEM_TIME_BASED_DEBOUNCE_THRSHOLD_DYN_CALL2 ==
  conditionfulfilled : Inport
  prefailed : Inport  Port=2
  prepassed : Inport  Port=3
  reseteventdebounce : Inport  Port=4
  DemDebounceBehavior : Inport  Port=5
  DemCounterFailedThreshold : Inport  Port=6
  DemCounterPassedThreshold : Inport  Port=7
  Enable : EnablePort
      settings: AttributesFormatString=StatesWhenEnabling = %<StatesWhenEnabling>
  AEMS_DEM_TIMEBASEDDEBOUNCE : AEMS_Standard_Library/SUB/AEMS_DEM_TIMEBASEDDEBOUNCE  Tag=[LIB]  eventid=Dem_EventId_Device2_Faulttype  sampletime=0.01
      settings: AttributesFormatString=|
      | %<MaskType>
      | EventId: %<eventid>
      | Sample time: %<sampletime>
  debouncevalue_for_failed : Outport
      settings: AttributesFormatString=<initial=%<InitialOutput>>\n<whendisabled=%<OutputWhenDisabled>>
  debouncevalue_for_passed : Outport  Port=2
      settings: AttributesFormatString=<initial=%<InitialOutput>>\n<whendisabled=%<OutputWhenDisabled>>
  failed : Outport  Port=3
      settings: AttributesFormatString=<initial=%<InitialOutput>>\n<whendisabled=%<OutputWhenDisabled>>
  passed : Outport  Port=4
      settings: AttributesFormatString=<initial=%<InitialOutput>>\n<whendisabled=%<OutputWhenDisabled>>
  wires:
  AEMS_DEM_TIMEBASEDDEBOUNCE/4 -> passed/1
  AEMS_DEM_TIMEBASEDDEBOUNCE/3 -> failed/1
  AEMS_DEM_TIMEBASEDDEBOUNCE/2 -> debouncevalue_for_passed/1
  AEMS_DEM_TIMEBASEDDEBOUNCE/1 -> debouncevalue_for_failed/1
  DemCounterFailedThreshold/1 -> AEMS_DEM_TIMEBASEDDEBOUNCE/5
  prefailed/1 -> AEMS_DEM_TIMEBASEDDEBOUNCE/2
  reseteventdebounce/1 -> AEMS_DEM_TIMEBASEDDEBOUNCE/7
  prepassed/1 -> AEMS_DEM_TIMEBASEDDEBOUNCE/3
  conditionfulfilled/1 -> AEMS_DEM_TIMEBASEDDEBOUNCE/1
  DemDebounceBehavior/1 -> AEMS_DEM_TIMEBASEDDEBOUNCE/4
  DemCounterPassedThreshold/1 -> AEMS_DEM_TIMEBASEDDEBOUNCE/6

== system AEMS_Standard_Library/SUB/AEMS_DEM_TIME_BASED_DEBOUNCE_THRSHOLD_DYN_8D/AEMS_DEM_TIME_BASED_DEBOUNCE_THRSHOLD_DYN_CALL3 ==
  conditionfulfilled : Inport
  prefailed : Inport  Port=2
  prepassed : Inport  Port=3
  reseteventdebounce : Inport  Port=4
  DemDebounceBehavior : Inport  Port=5
  DemCounterFailedThreshold : Inport  Port=6
  DemCounterPassedThreshold : Inport  Port=7
  Enable : EnablePort
      settings: AttributesFormatString=StatesWhenEnabling = %<StatesWhenEnabling>
  AEMS_DEM_TIMEBASEDDEBOUNCE : AEMS_Standard_Library/SUB/AEMS_DEM_TIMEBASEDDEBOUNCE  Tag=[LIB]  eventid=Dem_EventId_Device3_Faulttype  sampletime=0.01
      settings: AttributesFormatString=|
      | %<MaskType>
      | EventId: %<eventid>
      | Sample time: %<sampletime>
  debouncevalue_for_failed : Outport
      settings: AttributesFormatString=<initial=%<InitialOutput>>\n<whendisabled=%<OutputWhenDisabled>>
  debouncevalue_for_passed : Outport  Port=2
      settings: AttributesFormatString=<initial=%<InitialOutput>>\n<whendisabled=%<OutputWhenDisabled>>
  failed : Outport  Port=3
      settings: AttributesFormatString=<initial=%<InitialOutput>>\n<whendisabled=%<OutputWhenDisabled>>
  passed : Outport  Port=4
      settings: AttributesFormatString=<initial=%<InitialOutput>>\n<whendisabled=%<OutputWhenDisabled>>
  wires:
  AEMS_DEM_TIMEBASEDDEBOUNCE/4 -> passed/1
  AEMS_DEM_TIMEBASEDDEBOUNCE/3 -> failed/1
  AEMS_DEM_TIMEBASEDDEBOUNCE/2 -> debouncevalue_for_passed/1
  AEMS_DEM_TIMEBASEDDEBOUNCE/1 -> debouncevalue_for_failed/1
  DemCounterFailedThreshold/1 -> AEMS_DEM_TIMEBASEDDEBOUNCE/5
  prefailed/1 -> AEMS_DEM_TIMEBASEDDEBOUNCE/2
  reseteventdebounce/1 -> AEMS_DEM_TIMEBASEDDEBOUNCE/7
  prepassed/1 -> AEMS_DEM_TIMEBASEDDEBOUNCE/3
  conditionfulfilled/1 -> AEMS_DEM_TIMEBASEDDEBOUNCE/1
  DemDebounceBehavior/1 -> AEMS_DEM_TIMEBASEDDEBOUNCE/4
  DemCounterPassedThreshold/1 -> AEMS_DEM_TIMEBASEDDEBOUNCE/6

== system AEMS_Standard_Library/SUB/AEMS_DEM_TIME_BASED_DEBOUNCE_THRSHOLD_DYN_8D/AEMS_DEM_TIME_BASED_DEBOUNCE_THRSHOLD_DYN_CALL4 ==
  conditionfulfilled : Inport
  prefailed : Inport  Port=2
  prepassed : Inport  Port=3
  reseteventdebounce : Inport  Port=4
  DemDebounceBehavior : Inport  Port=5
  DemCounterFailedThreshold : Inport  Port=6
  DemCounterPassedThreshold : Inport  Port=7
  Enable : EnablePort
      settings: AttributesFormatString=StatesWhenEnabling = %<StatesWhenEnabling>
  AEMS_DEM_TIMEBASEDDEBOUNCE : AEMS_Standard_Library/SUB/AEMS_DEM_TIMEBASEDDEBOUNCE  Tag=[LIB]  eventid=Dem_EventId_Device4_Faulttype  sampletime=0.01
      settings: AttributesFormatString=|
      | %<MaskType>
      | EventId: %<eventid>
      | Sample time: %<sampletime>
  debouncevalue_for_failed : Outport
      settings: AttributesFormatString=<initial=%<InitialOutput>>\n<whendisabled=%<OutputWhenDisabled>>
  debouncevalue_for_passed : Outport  Port=2
      settings: AttributesFormatString=<initial=%<InitialOutput>>\n<whendisabled=%<OutputWhenDisabled>>
  failed : Outport  Port=3
      settings: AttributesFormatString=<initial=%<InitialOutput>>\n<whendisabled=%<OutputWhenDisabled>>
  passed : Outport  Port=4
      settings: AttributesFormatString=<initial=%<InitialOutput>>\n<whendisabled=%<OutputWhenDisabled>>
  wires:
  AEMS_DEM_TIMEBASEDDEBOUNCE/4 -> passed/1
  AEMS_DEM_TIMEBASEDDEBOUNCE/3 -> failed/1
  AEMS_DEM_TIMEBASEDDEBOUNCE/2 -> debouncevalue_for_passed/1
  AEMS_DEM_TIMEBASEDDEBOUNCE/1 -> debouncevalue_for_failed/1
  DemCounterFailedThreshold/1 -> AEMS_DEM_TIMEBASEDDEBOUNCE/5
  prefailed/1 -> AEMS_DEM_TIMEBASEDDEBOUNCE/2
  reseteventdebounce/1 -> AEMS_DEM_TIMEBASEDDEBOUNCE/7
  prepassed/1 -> AEMS_DEM_TIMEBASEDDEBOUNCE/3
  conditionfulfilled/1 -> AEMS_DEM_TIMEBASEDDEBOUNCE/1
  DemDebounceBehavior/1 -> AEMS_DEM_TIMEBASEDDEBOUNCE/4
  DemCounterPassedThreshold/1 -> AEMS_DEM_TIMEBASEDDEBOUNCE/6

== system AEMS_Standard_Library/SUB/AEMS_DEM_TIME_BASED_DEBOUNCE_THRSHOLD_DYN_8D/AEMS_DEM_TIME_BASED_DEBOUNCE_THRSHOLD_DYN_CALL5 ==
  conditionfulfilled : Inport
  prefailed : Inport  Port=2
  prepassed : Inport  Port=3
  reseteventdebounce : Inport  Port=4
  DemDebounceBehavior : Inport  Port=5
  DemCounterFailedThreshold : Inport  Port=6
  DemCounterPassedThreshold : Inport  Port=7
  Enable : EnablePort
      settings: AttributesFormatString=StatesWhenEnabling = %<StatesWhenEnabling>
  AEMS_DEM_TIMEBASEDDEBOUNCE : AEMS_Standard_Library/SUB/AEMS_DEM_TIMEBASEDDEBOUNCE  Tag=[LIB]  eventid=Dem_EventId_Device5_Faulttype  sampletime=0.01
      settings: AttributesFormatString=|
      | %<MaskType>
      | EventId: %<eventid>
      | Sample time: %<sampletime>
  debouncevalue_for_failed : Outport
      settings: AttributesFormatString=<initial=%<InitialOutput>>\n<whendisabled=%<OutputWhenDisabled>>
  debouncevalue_for_passed : Outport  Port=2
      settings: AttributesFormatString=<initial=%<InitialOutput>>\n<whendisabled=%<OutputWhenDisabled>>
  failed : Outport  Port=3
      settings: AttributesFormatString=<initial=%<InitialOutput>>\n<whendisabled=%<OutputWhenDisabled>>
  passed : Outport  Port=4
      settings: AttributesFormatString=<initial=%<InitialOutput>>\n<whendisabled=%<OutputWhenDisabled>>
  wires:
  AEMS_DEM_TIMEBASEDDEBOUNCE/4 -> passed/1
  AEMS_DEM_TIMEBASEDDEBOUNCE/3 -> failed/1
  AEMS_DEM_TIMEBASEDDEBOUNCE/2 -> debouncevalue_for_passed/1
  AEMS_DEM_TIMEBASEDDEBOUNCE/1 -> debouncevalue_for_failed/1
  DemCounterFailedThreshold/1 -> AEMS_DEM_TIMEBASEDDEBOUNCE/5
  prefailed/1 -> AEMS_DEM_TIMEBASEDDEBOUNCE/2
  reseteventdebounce/1 -> AEMS_DEM_TIMEBASEDDEBOUNCE/7
  prepassed/1 -> AEMS_DEM_TIMEBASEDDEBOUNCE/3
  conditionfulfilled/1 -> AEMS_DEM_TIMEBASEDDEBOUNCE/1
  DemDebounceBehavior/1 -> AEMS_DEM_TIMEBASEDDEBOUNCE/4
  DemCounterPassedThreshold/1 -> AEMS_DEM_TIMEBASEDDEBOUNCE/6

== system AEMS_Standard_Library/SUB/AEMS_DEM_TIME_BASED_DEBOUNCE_THRSHOLD_DYN_8D/AEMS_DEM_TIME_BASED_DEBOUNCE_THRSHOLD_DYN_CALL6 ==
  conditionfulfilled : Inport
  prefailed : Inport  Port=2
  prepassed : Inport  Port=3
  reseteventdebounce : Inport  Port=4
  DemDebounceBehavior : Inport  Port=5
  DemCounterFailedThreshold : Inport  Port=6
  DemCounterPassedThreshold : Inport  Port=7
  Enable : EnablePort
      settings: AttributesFormatString=StatesWhenEnabling = %<StatesWhenEnabling>
  AEMS_DEM_TIMEBASEDDEBOUNCE : AEMS_Standard_Library/SUB/AEMS_DEM_TIMEBASEDDEBOUNCE  Tag=[LIB]  eventid=Dem_EventId_Device6_Faulttype  sampletime=0.01
      settings: AttributesFormatString=|
      | %<MaskType>
      | EventId: %<eventid>
      | Sample time: %<sampletime>
  debouncevalue_for_failed : Outport
      settings: AttributesFormatString=<initial=%<InitialOutput>>\n<whendisabled=%<OutputWhenDisabled>>
  debouncevalue_for_passed : Outport  Port=2
      settings: AttributesFormatString=<initial=%<InitialOutput>>\n<whendisabled=%<OutputWhenDisabled>>
  failed : Outport  Port=3
      settings: AttributesFormatString=<initial=%<InitialOutput>>\n<whendisabled=%<OutputWhenDisabled>>
  passed : Outport  Port=4
      settings: AttributesFormatString=<initial=%<InitialOutput>>\n<whendisabled=%<OutputWhenDisabled>>
  wires:
  AEMS_DEM_TIMEBASEDDEBOUNCE/4 -> passed/1
  AEMS_DEM_TIMEBASEDDEBOUNCE/3 -> failed/1
  AEMS_DEM_TIMEBASEDDEBOUNCE/2 -> debouncevalue_for_passed/1
  AEMS_DEM_TIMEBASEDDEBOUNCE/1 -> debouncevalue_for_failed/1
  DemCounterFailedThreshold/1 -> AEMS_DEM_TIMEBASEDDEBOUNCE/5
  prefailed/1 -> AEMS_DEM_TIMEBASEDDEBOUNCE/2
  reseteventdebounce/1 -> AEMS_DEM_TIMEBASEDDEBOUNCE/7
  prepassed/1 -> AEMS_DEM_TIMEBASEDDEBOUNCE/3
  conditionfulfilled/1 -> AEMS_DEM_TIMEBASEDDEBOUNCE/1
  DemDebounceBehavior/1 -> AEMS_DEM_TIMEBASEDDEBOUNCE/4
  DemCounterPassedThreshold/1 -> AEMS_DEM_TIMEBASEDDEBOUNCE/6

== system AEMS_Standard_Library/SUB/AEMS_DEM_TIME_BASED_DEBOUNCE_THRSHOLD_DYN_8D/AEMS_DEM_TIME_BASED_DEBOUNCE_THRSHOLD_DYN_CALL7 ==
  conditionfulfilled : Inport
  prefailed : Inport  Port=2
  prepassed : Inport  Port=3
  reseteventdebounce : Inport  Port=4
  DemDebounceBehavior : Inport  Port=5
  DemCounterFailedThreshold : Inport  Port=6
  DemCounterPassedThreshold : Inport  Port=7
  Enable : EnablePort
      settings: AttributesFormatString=StatesWhenEnabling = %<StatesWhenEnabling>
  AEMS_DEM_TIMEBASEDDEBOUNCE : AEMS_Standard_Library/SUB/AEMS_DEM_TIMEBASEDDEBOUNCE  Tag=[LIB]  eventid=Dem_EventId_Device7_Faulttype  sampletime=0.01
      settings: AttributesFormatString=|
      | %<MaskType>
      | EventId: %<eventid>
      | Sample time: %<sampletime>
  debouncevalue_for_failed : Outport
      settings: AttributesFormatString=<initial=%<InitialOutput>>\n<whendisabled=%<OutputWhenDisabled>>
  debouncevalue_for_passed : Outport  Port=2
      settings: AttributesFormatString=<initial=%<InitialOutput>>\n<whendisabled=%<OutputWhenDisabled>>
  failed : Outport  Port=3
      settings: AttributesFormatString=<initial=%<InitialOutput>>\n<whendisabled=%<OutputWhenDisabled>>
  passed : Outport  Port=4
      settings: AttributesFormatString=<initial=%<InitialOutput>>\n<whendisabled=%<OutputWhenDisabled>>
  wires:
  AEMS_DEM_TIMEBASEDDEBOUNCE/4 -> passed/1
  AEMS_DEM_TIMEBASEDDEBOUNCE/3 -> failed/1
  AEMS_DEM_TIMEBASEDDEBOUNCE/2 -> debouncevalue_for_passed/1
  AEMS_DEM_TIMEBASEDDEBOUNCE/1 -> debouncevalue_for_failed/1
  DemCounterFailedThreshold/1 -> AEMS_DEM_TIMEBASEDDEBOUNCE/5
  prefailed/1 -> AEMS_DEM_TIMEBASEDDEBOUNCE/2
  reseteventdebounce/1 -> AEMS_DEM_TIMEBASEDDEBOUNCE/7
  prepassed/1 -> AEMS_DEM_TIMEBASEDDEBOUNCE/3
  conditionfulfilled/1 -> AEMS_DEM_TIMEBASEDDEBOUNCE/1
  DemDebounceBehavior/1 -> AEMS_DEM_TIMEBASEDDEBOUNCE/4
  DemCounterPassedThreshold/1 -> AEMS_DEM_TIMEBASEDDEBOUNCE/6

== system AEMS_Standard_Library/SUB/AEMS_DEM_TIME_BASED_DEBOUNCE_THRSHOLD_DYN_8D/AEMS_DEM_TIME_BASED_DEBOUNCE_THRSHOLD_DYN_CALL8 ==
  conditionfulfilled : Inport
  prefailed : Inport  Port=2
  prepassed : Inport  Port=3
  reseteventdebounce : Inport  Port=4
  DemDebounceBehavior : Inport  Port=5
  DemCounterFailedThreshold : Inport  Port=6
  DemCounterPassedThreshold : Inport  Port=7
  Enable : EnablePort
      settings: AttributesFormatString=StatesWhenEnabling = %<StatesWhenEnabling>
  AEMS_DEM_TIMEBASEDDEBOUNCE : AEMS_Standard_Library/SUB/AEMS_DEM_TIMEBASEDDEBOUNCE  Tag=[LIB]  eventid=Dem_EventId_Device8_Faulttype  sampletime=0.01
      settings: AttributesFormatString=|
      | %<MaskType>
      | EventId: %<eventid>
      | Sample time: %<sampletime>
  debouncevalue_for_failed : Outport
      settings: AttributesFormatString=<initial=%<InitialOutput>>\n<whendisabled=%<OutputWhenDisabled>>
  debouncevalue_for_passed : Outport  Port=2
      settings: AttributesFormatString=<initial=%<InitialOutput>>\n<whendisabled=%<OutputWhenDisabled>>
  failed : Outport  Port=3
      settings: AttributesFormatString=<initial=%<InitialOutput>>\n<whendisabled=%<OutputWhenDisabled>>
  passed : Outport  Port=4
      settings: AttributesFormatString=<initial=%<InitialOutput>>\n<whendisabled=%<OutputWhenDisabled>>
  wires:
  AEMS_DEM_TIMEBASEDDEBOUNCE/4 -> passed/1
  AEMS_DEM_TIMEBASEDDEBOUNCE/3 -> failed/1
  AEMS_DEM_TIMEBASEDDEBOUNCE/2 -> debouncevalue_for_passed/1
  AEMS_DEM_TIMEBASEDDEBOUNCE/1 -> debouncevalue_for_failed/1
  DemCounterFailedThreshold/1 -> AEMS_DEM_TIMEBASEDDEBOUNCE/5
  prefailed/1 -> AEMS_DEM_TIMEBASEDDEBOUNCE/2
  reseteventdebounce/1 -> AEMS_DEM_TIMEBASEDDEBOUNCE/7
  prepassed/1 -> AEMS_DEM_TIMEBASEDDEBOUNCE/3
  conditionfulfilled/1 -> AEMS_DEM_TIMEBASEDDEBOUNCE/1
  DemDebounceBehavior/1 -> AEMS_DEM_TIMEBASEDDEBOUNCE/4
  DemCounterPassedThreshold/1 -> AEMS_DEM_TIMEBASEDDEBOUNCE/6

== system AEMS_Standard_Library/SUB/AEMS_SORT_MEDIAN/Odd ==
  Vector_size : Inport
  Sorted_vector : Inport  Port=2
  Action Port : ActionPort
  Add : Sum  OutDataTypeStr=Inherit: Inherit via back propagation
  Constant : Constant  OutDataTypeStr=uint8
  Constant1 : Constant  Value=2  OutDataTypeStr=uint8
  Divide : Product  Inputs=*/  OutDataTypeStr=Inherit: Inherit via back propagation
  Selector : Selector  IndexMode=Zero-based  InputPortWidth=N  IndexOptions=Index vector (port)  Indices=[1 3]  OutputSizes=1
  Median_Odd : Outport
  wires:
  Vector_size/1 -> Add/1
  Constant/1 -> Add/2
  Add/1 -> Divide/1
  Constant1/1 -> Divide/2
  Sorted_vector/1 -> Selector/1
  Divide/1 -> Selector/2
  Selector/1 -> Median_Odd/1
